simulink model "problem_7"  (R2020b)
settings: Solver=VariableStepAuto  StartTime=0.0  StopTime=10.0  RelTol=1e-3
settings Model: Creator=k.Raviteja  LastModifiedBy=k.Raviteja

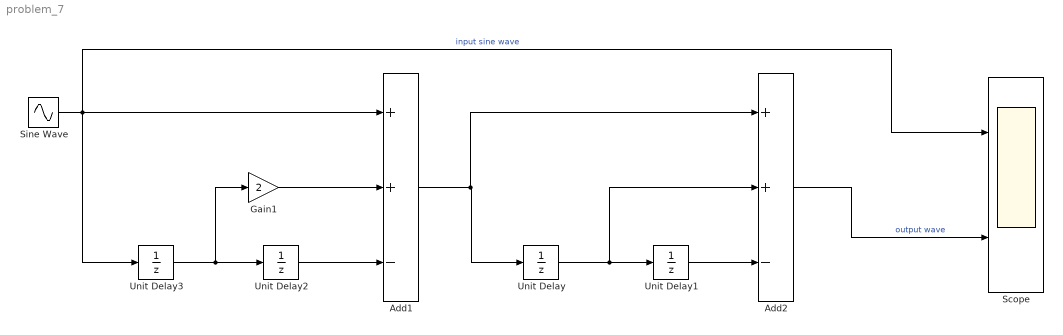
== system problem_7 ==
  Add1 : Sum  Inputs=++-
  Add2 : Sum  Inputs=++-
  Gain1 : Gain  Gain=2
  Scope : Scope  NumInputPorts=2
  Sine Wave : Sin  SampleTime=0
  Unit Delay{,1..3} (4 alike) : UnitDelay  SampleTime=-1  HasFrameUpgradeWarning=on
  wires:
  Unit Delay3/1 -> Gain1/1, Unit Delay2/1
  Unit Delay/1 -> Add2/2, Unit Delay1/1
  Sine Wave/1 -> Unit Delay3/1, Scope/1, Add1/1  "input sine wave"
  Add1/1 -> Add2/1, Unit Delay/1
  Unit Delay2/1 -> Add1/3
  Gain1/1 -> Add1/2
  Unit Delay1/1 -> Add2/3
  Add2/1 -> Scope/2  "output wave"
